simulink model "IMmathematicalmodelfluxlinkage"  (R2018b)
settings: Solver=ode4  StartTime=0.0  StopTime=1  RelTol=1e-3
values from neighbouring files (symbols this model uses):
  B = 0.001    [inductionmotordata.m]
  D = Xss*Xrr-Xm^2    (= 2336.07942961)    [inductionmotordata.m]
  J = 0.004    [inductionmotordata.m]
  Lm = 280/(2*pi*f)    (= 0.891267681315)    [inductionmotordata.m]
  p = 2    [inductionmotordata.m]
  R1 = 6.76    [inductionmotordata.m]
  R2 = 2.41    [inductionmotordata.m]
  wb = 2*pi*f    (= 314.159265359)    [inductionmotordata.m]
  ws = wb*2/p    (= 314.159265359)    [inductionmotordata.m]
  Xm = 1.5*wb*Lm    (= 420)    [inductionmotordata.m]
  Xrr = wb*(L2+1.5*Lm)    (= 422.7719)    [inductionmotordata.m]
  Xss = wb*(L1+1.5*Lm)    (= 422.7719)    [inductionmotordata.m]
undefined symbols (not defined in the file or in its folder): i
libraries: powerlib x7
settings Model: Creator=BALA  LastModifiedBy=Bala

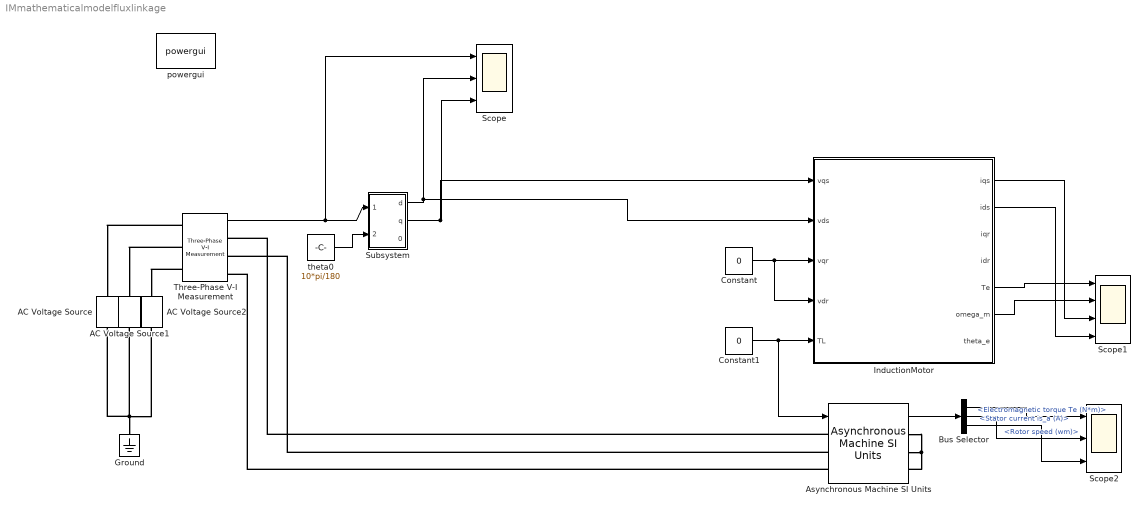
== system IMmathematicalmodelfluxlinkage ==
  AC Voltage Source : powerlib/Electrical Sources/AC Voltage Source  Amplitude=325  Phase=10  Frequency=50  SampleTime=0  Measurements=None  BusType=swing  Pref=10e3  Qref=0  Qmin=-inf  Qmax=+inf
  AC Voltage Source1 : powerlib/Electrical Sources/AC Voltage Source  Amplitude=325  Phase=-110  Frequency=50  SampleTime=0  Measurements=None  BusType=swing  Pref=10e3  Qref=0  Qmin=-inf  Qmax=+inf
  AC Voltage Source2 : powerlib/Electrical Sources/AC Voltage Source  Amplitude=325  Phase=130  Frequency=50  SampleTime=0  Measurements=None  BusType=swing  Pref=10e3  Qref=0  Qmin=-inf  Qmax=+inf
  Asynchronous Machine SI Units : powerlib/Machines/Asynchronous Machine SI Units  RotorType=Wound  PresetModel=No  MechanicalLoad=Torque Tm  ShowDetailedParameters=on  ReferenceFrame=Rotor  Units=SI  MeasurementBus=off  NominalParameters=[2152 415 50]  Stator=[7.76 0.00882]  Rotor=[5.41 0.00882]  Cage1=[0.4155 0.002066]  Cage2=[0.4168 0.0003495]  Lm=0.8926  Mechanical=[0.004 0.005879 1]  PolePairs=2  InitialConditions=[1 0 0 0 0 0 0 0]  SimulateSaturation=off  Saturation=[14.03593122, 27.81365428, 53.79336849, 72.68890987, 97.98006896, 148.6815601, 215.7428561, 302.9841135, 428.7778367 ; 230, 322, 414, 460, 506, 552, 598, 644, 690]  LoadFlowParameters=1492000  TsPowergui=0  TsBlock=-1  IterativeModel=Trapezoidal non iterative  IterativeDiscreteModel=Trapezoidal non iterative  Pmec=1.492e+006
  Bus Selector : BusSelector  OutputSignals=Mechanical.Electromagnetic torque Te (N*m),Mechanical.Rotor speed (wm),Stator measurements.Stator current is_a (A)
  Constant : Constant  Value=0
  Constant1 : Constant  Value=0
  Ground : powerlib/Elements/Ground  LConnTagsString=a
  InductionMotor : Subsystem
  Scope : Scope  NumInputPorts=3
  Scope1 : Scope  NumInputPorts=4
  Scope2 : Scope  NumInputPorts=3
  Subsystem : Subsystem
  Three-Phase V-I Measurement : powerlib/Measurements/Three-Phase V-I Measurement  VoltageMeasurement=phase-to-ground  SetLabelV=off  LabelV=Vabc  Vpu=off  VpuLL=off  CurrentMeasurement=no  SetLabelI=off  LabelI=Iabc  Ipu=off  Pbase=100e6  Vbase=500e3  OutputType=Complex  PhasorSimulation=off  PSBequivalent=0
  powergui : powerlib/powergui  Priority=1  SimulationMode=Discrete  SampleTime=5e-6  frequency=60  Iterations=50  frequencyindice=50  Pbase=100e6  ErrMax=1e-4  UnitsV=kV  UnitsW=MW  buscounter=0  FunctionMessages=off  echomessages=off  EnableUseOfTLC=off  CurrentSourceSwitches=off  DisableSnubberDevices=off  DisableRonSwitches=off  DisableVfSwitches=off  DisplayEquations=off  SolverType=Tustin/Backward Euler (TBE)  Interpol=off  ExternalGateDelay=off  methode=off  Ts=100  x0status=blocks  SPID=off  SwTol=0  HookPort=off  RestoreLinks=warning  ResistiveCurrentMeasurement=off  Frange=[0:2:500]  Ylog=off  Xlog=on  ShowGrid=off  save=off  variable=ZData  structure=0  ZoomFFT=off  StartTime=0.0  cycles=1  DisplayStyle=1  fundamental=60  FreqAxis=off  MaxFrequency=1000  frequencyindicesteady=1  RmsSteady=1  display=off
  theta0 : Constant  Value=10*pi/180
  wires:
  Constant/1 -> InductionMotor/4(vdr), InductionMotor/3(vqr)
  Constant1/1 -> Asynchronous Machine SI Units/1, InductionMotor/5(TL)
  Three-Phase V-I Measurement/1 -> Subsystem/1(ABC), Scope/1
  theta0/1 -> Subsystem/2(theta0)
  Subsystem/1(d) -> InductionMotor/2(vds), Scope/2
  Subsystem/2(q) -> InductionMotor/1(vqs), Scope/3
  InductionMotor/5(Te) -> Scope1/1
  InductionMotor/6(omega_m) -> Scope1/2
  Asynchronous Machine SI Units/1 -> Bus Selector/1
  Bus Selector/1 -> Scope2/1  "<Electromagnetic torque Te (N*m)>"
  Bus Selector/2 -> Scope2/2  "<Rotor speed (wm)>"
  Bus Selector/3 -> Scope2/3  "<Stator current is_a (A)>"
  InductionMotor/1(iqs) -> Scope1/3
  InductionMotor/2(ids) -> Scope1/4
  connections:
  AC Voltage Source2/LConn1 -- AC Voltage Source1/LConn1 -- AC Voltage Source/LConn1 -- Ground/LConn1
  Three-Phase V-I Measurement/LConn1 -- AC Voltage Source/RConn1
  Three-Phase V-I Measurement/LConn3 -- AC Voltage Source2/RConn1
  Three-Phase V-I Measurement/LConn2 -- AC Voltage Source1/RConn1
  Asynchronous Machine SI Units/LConn1 -- Three-Phase V-I Measurement/RConn1
  Asynchronous Machine SI Units/LConn2 -- Three-Phase V-I Measurement/RConn2
  Asynchronous Machine SI Units/LConn3 -- Three-Phase V-I Measurement/RConn3
  Asynchronous Machine SI Units/RConn1 -- Asynchronous Machine SI Units/RConn2 -- Asynchronous Machine SI Units/RConn3

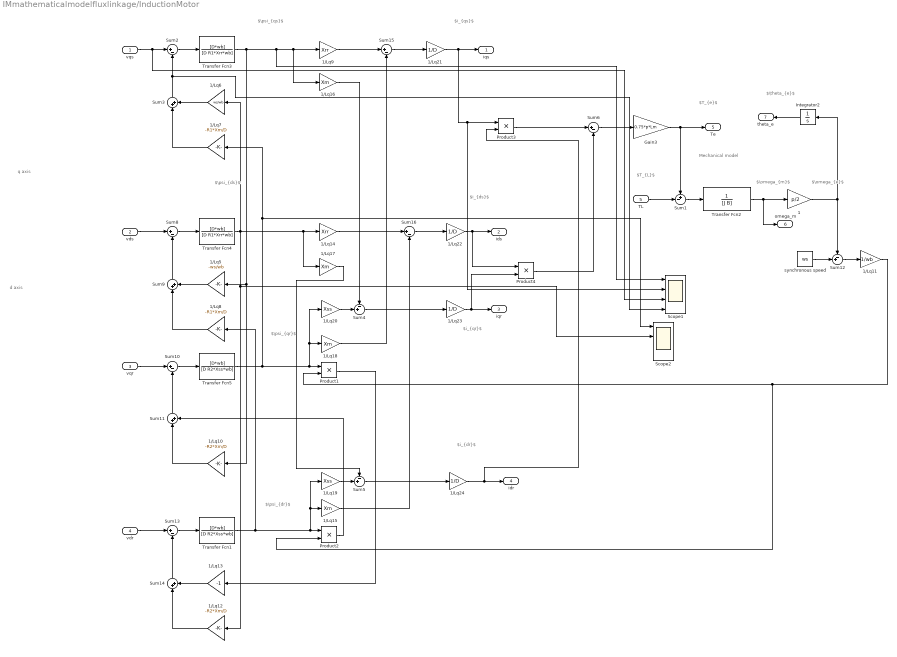
== system IMmathematicalmodelfluxlinkage/InductionMotor ==
  note: Mechanical model
  note: $i_{qs}$
  note: $i_{ds}$
  note: $T_{e}$
  note: d axis
  note: q axis
  note: $\omega_{m}$
  note: $\omega_{e}$
  note: $\theta_{e}$
  note: $T_{L}$
  note: $\psi_{qs}$
  note: $\psi_{ds}$
  note: $\psi_{qr}$
  note: $\psi_{dr}$
  note: $i_{qr}$
  note: $i_{dr}$
  vqs : Inport
  vds : Inport  Port=2
  vqr : Inport  Port=3
  vdr : Inport  Port=4
  TL : Inport  Port=5
  "  1" : Gain  Gain=p/2  OutDataTypeStr=Inherit: Same as input  ParamDataTypeStr=Inherit: Same as input
  1/Lq10 : Gain  Gain=-R2*Xm/D  SaturateOnIntegerOverflow=on  OutDataTypeStr=Inherit: Same as input  ParamDataTypeStr=Inherit: Same as input
  1/Lq11 : Gain  Gain=1/wb  SaturateOnIntegerOverflow=on  OutDataTypeStr=Inherit: Same as input  ParamDataTypeStr=Inherit: Same as input
  1/Lq12 : Gain  Gain=-R2*Xm/D  SaturateOnIntegerOverflow=on  OutDataTypeStr=Inherit: Same as input  ParamDataTypeStr=Inherit: Same as input
  1/Lq13 : Gain  Gain=-1  SaturateOnIntegerOverflow=on  OutDataTypeStr=Inherit: Same as input  ParamDataTypeStr=Inherit: Same as input
  1/Lq14 : Gain  Gain=Xrr  SaturateOnIntegerOverflow=on  OutDataTypeStr=Inherit: Same as input  ParamDataTypeStr=Inherit: Same as input
  1/Lq{15..18} (4 alike) : Gain  Gain=Xm  SaturateOnIntegerOverflow=on  OutDataTypeStr=Inherit: Same as input  ParamDataTypeStr=Inherit: Same as input
  1/Lq19 : Gain  Gain=Xss  SaturateOnIntegerOverflow=on  OutDataTypeStr=Inherit: Same as input  ParamDataTypeStr=Inherit: Same as input
  1/Lq20 : Gain  Gain=Xss  SaturateOnIntegerOverflow=on  OutDataTypeStr=Inherit: Same as input  ParamDataTypeStr=Inherit: Same as input
  1/Lq{21..24} (4 alike) : Gain  Gain=1/D  SaturateOnIntegerOverflow=on  OutDataTypeStr=Inherit: Same as input  ParamDataTypeStr=Inherit: Same as input
  1/Lq5 : Gain  Gain=-ws/wb  SaturateOnIntegerOverflow=on  OutDataTypeStr=Inherit: Same as input  ParamDataTypeStr=Inherit: Same as input
  1/Lq6 : Gain  Gain=ws/wb  SaturateOnIntegerOverflow=on  OutDataTypeStr=Inherit: Same as input  ParamDataTypeStr=Inherit: Same as input
  1/Lq7 : Gain  Gain=-R1*Xm/D  SaturateOnIntegerOverflow=on  OutDataTypeStr=Inherit: Same as input  ParamDataTypeStr=Inherit: Same as input
  1/Lq8 : Gain  Gain=-R1*Xm/D  SaturateOnIntegerOverflow=on  OutDataTypeStr=Inherit: Same as input  ParamDataTypeStr=Inherit: Same as input
  1/Lq9 : Gain  Gain=Xrr  SaturateOnIntegerOverflow=on  OutDataTypeStr=Inherit: Same as input  ParamDataTypeStr=Inherit: Same as input
  Gain3 : Gain  Gain=0.75*p*Lm  SaturateOnIntegerOverflow=on  OutDataTypeStr=Inherit: Same as input  ParamDataTypeStr=Inherit: Same as input
  Integrator2 : Integrator
  Product{1..4} (4 alike) : Product  SaturateOnIntegerOverflow=on  InputSameDT=on  OutDataTypeStr=Inherit: Same as first input
  Scope1 : Scope  NumInputPorts=4
  Scope2 : Scope  NumInputPorts=4
  Sum1 : Sum  Inputs=+-|  SaturateOnIntegerOverflow=on  InputSameDT=on  OutDataTypeStr=Inherit: Same as first input
  Sum{2,6,8,10,13,15..16} (7 alike) : Sum  Inputs=|+-  SaturateOnIntegerOverflow=on  InputSameDT=on  OutDataTypeStr=Inherit: Same as first input
  Sum{3,9,11,14} (4 alike) : Sum  Inputs=|++  SaturateOnIntegerOverflow=on  InputSameDT=on  OutDataTypeStr=Inherit: Same as first input
  Sum12 : Sum  Inputs=-+|  SaturateOnIntegerOverflow=on  InputSameDT=on  OutDataTypeStr=Inherit: Same as first input
  Sum4 : Sum  Inputs=-+|  SaturateOnIntegerOverflow=on  InputSameDT=on  OutDataTypeStr=Inherit: Same as first input
  Sum5 : Sum  Inputs=-+|  SaturateOnIntegerOverflow=on  InputSameDT=on  OutDataTypeStr=Inherit: Same as first input
  Transfer Fcn1 : TransferFcn  Numerator=[D*wb]  Denominator=[D R2*Xss*wb]
  Transfer Fcn2 : TransferFcn  Denominator=[J B]
  Transfer Fcn3 : TransferFcn  Numerator=[D*wb]  Denominator=[D R1*Xrr*wb]
  Transfer Fcn4 : TransferFcn  Numerator=[D*wb]  Denominator=[D R1*Xrr*wb]
  Transfer Fcn5 : TransferFcn  Numerator=[D*wb]  Denominator=[D R2*Xss*wb]
  synchronous speed : Constant  Value=ws
  iqs : Outport
  ids : Outport  Port=2
  iqr : Outport  Port=3
  idr : Outport  Port=4
  Te : Outport  Port=5
  omega_m : Outport  Port=6
  theta_e : Outport  Port=7
  wires:
  Integrator2/1 -> theta_e/1
  Gain3/1 -> Sum1/1, Te/1
  Transfer Fcn2/1 -> omega_m/1, "  1"/1
  "  1"/1 -> Integrator2/1, Sum12/1
  Sum1/1 -> Transfer Fcn2/1
  TL/1 -> Sum1/2
  vqs/1 -> Scope1/3, Sum2/1
  1/Lq7/1 -> Sum3/1
  1/Lq6/1 -> Sum3/2
  Sum3/1 -> Scope1/4, Sum2/2
  Sum2/1 -> Transfer Fcn3/1
  Sum8/1 -> Transfer Fcn4/1
  Sum9/1 -> Sum8/2
  1/Lq5/1 -> Sum9/2
  1/Lq8/1 -> Sum9/1
  vds/1 -> Sum8/1
  Transfer Fcn3/1 -> Scope1/1, 1/Lq16/1, 1/Lq9/1, 1/Lq10/1, 1/Lq5/1
  Transfer Fcn4/1 -> 1/Lq17/1, 1/Lq14/1, Scope2/2, 1/Lq12/1, 1/Lq6/1
  vqr/1 -> Sum10/1
  1/Lq10/1 -> Sum11/1
  Product2/1 -> Sum11/2
  Sum11/1 -> Sum10/2
  Sum10/1 -> Transfer Fcn5/1
  synchronous speed/1 -> Sum12/2
  Sum12/1 -> 1/Lq11/1
  1/Lq11/1 -> Product1/2, Product2/2
  Sum13/1 -> Transfer Fcn1/1
  Sum14/1 -> Sum13/2
  1/Lq13/1 -> Sum14/2
  1/Lq12/1 -> Sum14/1
  vdr/1 -> Sum13/1
  Transfer Fcn5/1 -> 1/Lq7/1, Scope2/1, 1/Lq18/1, 1/Lq20/1, Product1/1
  Transfer Fcn1/1 -> 1/Lq8/1, Product2/1, 1/Lq19/1, 1/Lq15/1
  Product1/1 -> 1/Lq13/1
  1/Lq9/1 -> Sum15/1
  1/Lq18/1 -> Sum15/2
  Sum15/1 -> 1/Lq21/1
  1/Lq21/1 -> Scope1/2, Product3/1, iqs/1
  1/Lq14/1 -> Sum16/1
  1/Lq15/1 -> Sum16/2
  Sum16/1 -> 1/Lq22/1
  1/Lq22/1 -> Product4/1, ids/1
  1/Lq20/1 -> Sum4/2
  1/Lq16/1 -> Sum4/1
  Sum4/1 -> 1/Lq23/1
  1/Lq23/1 -> Product4/2, iqr/1
  1/Lq19/1 -> Sum5/2
  Sum5/1 -> 1/Lq24/1
  1/Lq24/1 -> Product3/2, idr/1
  1/Lq17/1 -> Sum5/1
  Product3/1 -> Sum6/1
  Product4/1 -> Sum6/2
  Sum6/1 -> Gain3/1

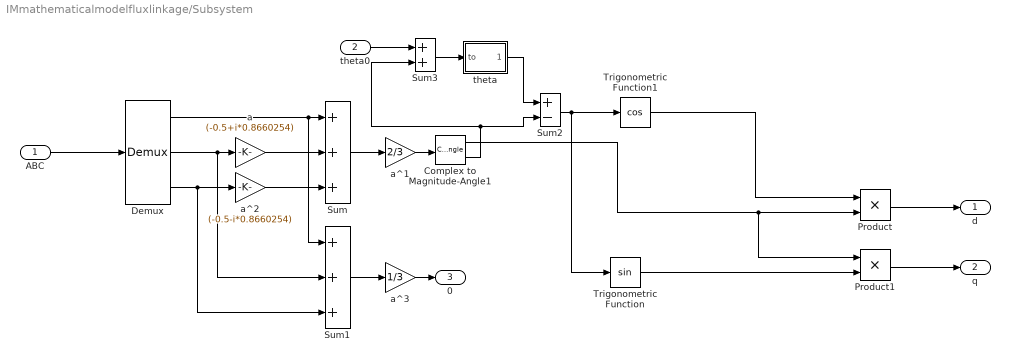
== system IMmathematicalmodelfluxlinkage/Subsystem ==
  ABC : Inport
  theta0 : Inport  Port=2
  Complex to Magnitude-Angle1 : ComplexToMagnitudeAngle
  Demux : Demux  Outputs=3
  Product : Product
  Product1 : Product
  Sum : Sum  Inputs=+++
  Sum1 : Sum  Inputs=+++
  Sum2 : Sum  Inputs=+-
  Sum3 : Sum
  Trigonometric Function : Trigonometry
  Trigonometric Function1 : Trigonometry  Operator=cos
  a : Gain  Gain=(-0.5+i*0.8660254)
  a^1 : Gain  Gain=2/3
  a^2 : Gain  Gain=(-0.5-i*0.8660254)
  a^3 : Gain  Gain=1/3
  theta : Subsystem
  d : Outport
  q : Outport  Port=2
  0 : Outport  Port=3
  wires:
  Demux/3 -> Sum1/3, a^2/1
  Demux/2 -> Sum1/2, a/1
  a/1 -> Sum/2
  Sum1/1 -> a^3/1
  a^2/1 -> Sum/3
  Sum/1 -> a^1/1
  a^3/1 -> 0/1
  ABC/1 -> Demux/1
  Trigonometric Function/1 -> Product1/2
  Product/1 -> d/1
  Product1/1 -> q/1
  Demux/1 -> Sum1/1, Sum/1
  a^1/1 -> Complex to Magnitude-Angle1/1
  Sum2/1 -> Trigonometric Function/1, Trigonometric Function1/1
  Trigonometric Function1/1 -> Product/1
  Complex to Magnitude-Angle1/1 -> Product1/1, Product/2
  theta/1(theta) -> Sum2/1
  Complex to Magnitude-Angle1/2 -> Sum2/2, Sum3/2
  Sum3/1 -> theta/1(to)
  theta0/1 -> Sum3/1

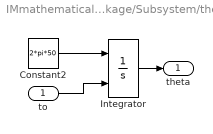
== system IMmathematicalmodelfluxlinkage/Subsystem/theta ==
  to : Inport
  Constant2 : Constant  Value=2*pi*50
  Integrator : Integrator  InitialConditionSource=external  UpperSaturationLimit=pi  LowerSaturationLimit=-pi
  theta : Outport
  wires:
  Constant2/1 -> Integrator/1
  Integrator/1 -> theta/1
  to/1 -> Integrator/2
